simulink model "Robot_10"  (R2023a)
settings: Solver=VariableStepAuto  StartTime=0.0  StopTime=15  RelTol=1e-3
values from neighbouring files (symbols this model uses):
  L2 = 2.3    [Jacobienne.m]    (also in Tracking.m)
undefined symbols (not defined in the file or in its folder): X, Y, Z
libraries: sm_lib x31, nesl_utility x11, slpidlib x2, SignalEditorBlockLib x2
(part 2 of 2)

== matlab function Robot_10/Jacobienne ==
  data: u input; w1 output; w2 output; w3 output; x output; y output; z output
function [w1, w2, w3, x, y, z] = fcn(u)

 q1 = u(1);

 q2 = u(2);

 dx = u(3);

 dy = u(4);

 dz = u(5);

 %-------------------------------------------------------------------------
 L1 = 0 ;

 L2 = 2.3;

 L3 = 4.5;

 rho = L3;

 teta = q1;

 phi = q2 + pi/2;

 x = rho*cos(phi)*cos(teta);

 y = rho*cos(phi)*sin(teta);

 z = rho*cos(phi);   

%  x = -L3*cos(q1)*sin(q2);
% 
%  y = -L3*sin(q1)*sin(q2);
% 
%  z = L3*cos(q2); 
%-------------------------------------------------------------------------

 J = [-rho*cos(phi)*sin(teta) -rho*sin(phi)*cos(teta) cos(phi)*cos(teta); rho*cos(phi)*cos(teta) -rho*sin(phi)*sin(teta) cos(phi)*sin(teta); 0 rho*cos(phi) sin(phi)];

 J_inv = inv(J);

%-------------------------------------------------------------------------

vitesse = [ dx ; dy ; dz ];
%vitesse = [(:), dy(:), dz(:)]';


w = J_inv*vitesse;

w1 = w(1);

w2 = w(2);

w3 = w(3);

end



%----------------------------------------------------------------------------------------------



% function [w1, w2, w3, x, y, z] = fcn(u)
% 
%     q1 = u(1);
%     q2 = u(2);
% 
%     dx = u(3);
%     dy = u(4);
%     dz = u(5);
% 
%     %-------------------------------------------------------------------------
%     L1 = 0 ;
%     L2 = 2.3;
%     L3 = 4.5;
% 
%     rho = L3;
% 
%     teta = q1;
%     phi = q2 + pi/2;
% 
%     x = rho*cos(phi)*cos(teta);
%     y = rho*cos(phi)*sin(teta);
%     z = rho*cos(phi);
% 
%     J = [-rho*cos(phi)*sin(teta) -rho*sin(phi)*cos(teta) cos(phi)*cos(teta);
%          rho*cos(phi)*cos(teta) -rho*sin(phi)*sin(teta) cos(phi)*sin(teta);
%          0 rho*cos(phi) sin(phi)];
% 
%     J_inv = inv(J);
% 
%     %-------------------------------------------------------------------------
% 
%     % vitesse = [dx ; dy ; dz];
%     vitesse = [dx(:), dy(:), dz(:)].';
% 
%     w = J_inv * vitesse.';
% 
%     w1 = w(1,:);
%     w2 = w(2,:);
%     w3 = w(3,:);
% 
% end
